simulink model "Lab_2"  (R2022b)
settings: Solver=VariableStepAuto  StartTime=0.0  StopTime=10.0  RelTol=1e-3
settings Model: Creator=adlercohen  LastModifiedBy=adlercohen

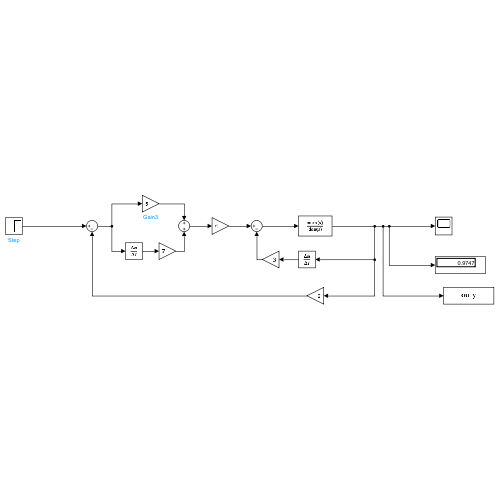
[thumbnail: Simulink's stored preview of the top-level diagram]
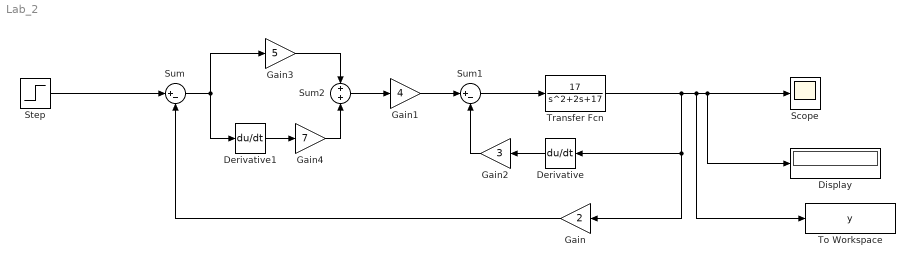
== system Lab_2 ==
  Derivative : Derivative
  Derivative1 : Derivative
  Display : Display
  Gain : Gain  Gain=2
  Gain1 : Gain  Gain=4
  Gain2 : Gain  Gain=3
  Gain3 : Gain  Gain=5
  Gain4 : Gain  Gain=7
  Scope : Scope
  Step : Step  Time=0  After=2  SampleTime=0
  Sum : Sum  Inputs=|+-
  Sum1 : Sum  Inputs=|+-
  Sum2 : Sum  Inputs=+|+
  To Workspace : ToWorkspace  VariableName=y  SampleTime=-1
  Transfer Fcn : TransferFcn  Numerator=[17]  Denominator=[1 2 17]
  wires:
  Gain2/1 -> Sum1/2
  Sum1/1 -> Transfer Fcn/1
  Transfer Fcn/1 -> Derivative/1, Gain/1, To Workspace/1, Display/1, Scope/1
  Derivative/1 -> Gain2/1
  Step/1 -> Sum/1
  Gain1/1 -> Sum1/1
  Gain/1 -> Sum/2
  Sum2/1 -> Gain1/1
  Derivative1/1 -> Gain4/1
  Gain4/1 -> Sum2/2
  Sum/1 -> Derivative1/1, Gain3/1
  Gain3/1 -> Sum2/1
